simulink model "opv_receiver_HDL_coder_input_ISRO_Paper"  (R2023a)
settings: Solver=FixedStepDiscrete  StartTime=0.0  StopTime=0.01*(samples_per_frame/sample_rate)  RelTol=1e-3
values from neighbouring files (symbols this model uses):
  bit_rate = bits_per_symbol*symbol_rate    (= 54200)    [opv.m]
  bits_per_symbol = 2    [opv.m]
  carrier_frequency = carrier_frequency_multiple_ceil*(orthogonal_frequency)    [opv.m]
  device_clock = 245.76e6    (= 245760000)    [opv.m]
  orthogonal_frequency = 1/(4*bit_period)    (= 13550)    [opv.m]
  symbol_rate = 27100    [opv.m]
libraries: dspsrcs4 x4, simulink_extras x2, hdlsllib x1, commsrccod2 x1, dsphdlsigops2 x1, commrandsrc3 x1
settings Model: Creator=matt  LastModifiedBy=matt
settings OptimizationCC: BlockReduction=off  ConditionallyExecuteInputs=off  DefaultParameterBehavior=Inlined
settings DebuggingCC: AlgebraicLoopMsg=error
settings HardwareCC: ProdBitPerPointer=32  ProdBitPerSizeT=32  ProdBitPerPtrDiffT=32  ProdLargestAtomicFloat=None  ProdIntDivRoundTo=Undefined  ProdEndianess=Unspecified  ProdWordSize=32  ProdHWDeviceType=ASIC/FPGA->ASIC/FPGA  TargetBitPerLong=64  TargetBitPerPointer=64  TargetBitPerSizeT=64  TargetBitPerPtrDiffT=64  TargetLongLongMode=on  TargetIntDivRoundTo=Zero  TargetEndianess=LittleEndian  TargetWordSize=64  TargetHWDeviceType=Custom Processor->MATLAB Host Computer  ProdEqTarget=off

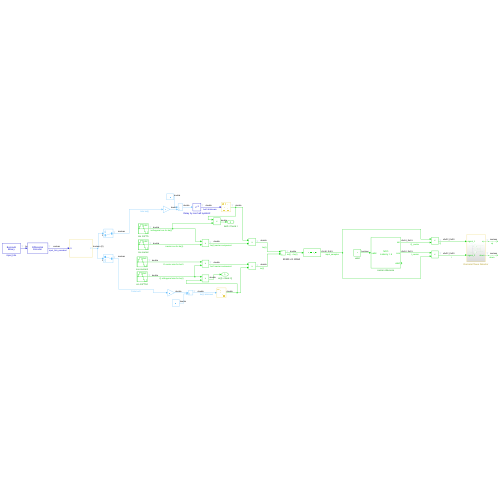
[thumbnail: Simulink's stored preview of the top-level diagram]
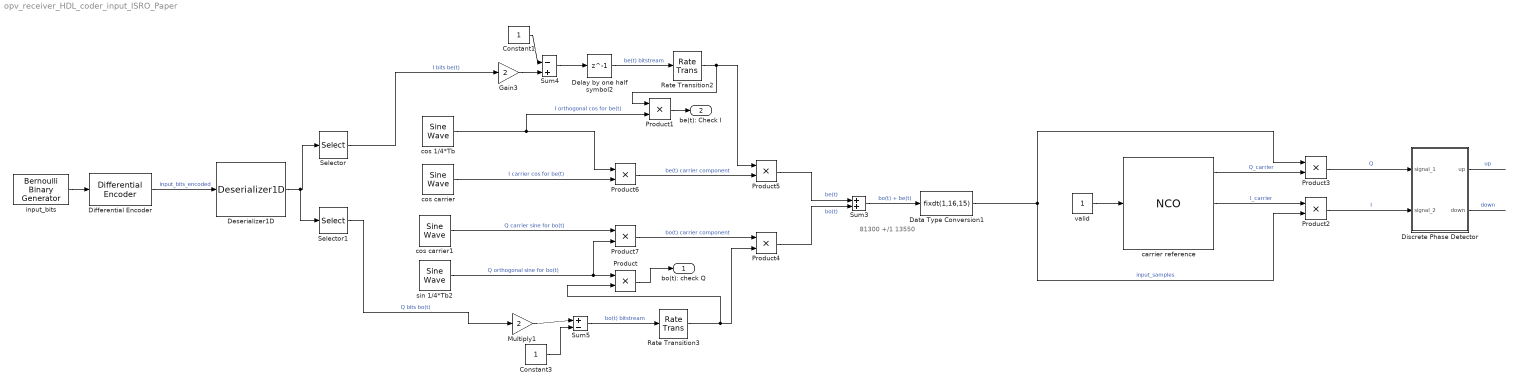
== system opv_receiver_HDL_coder_input_ISRO_Paper ==
  note: 81300 +/1 13550
  Constant1 : Constant  OutDataTypeStr=double  SampleTime=1/symbol_rate
  Constant3 : Constant  OutDataTypeStr=double  SampleTime=1/symbol_rate
  Data Type Conversion1 : DataTypeConversion  OutDataTypeStr=fixdt(1,16,15)  SaturateOnIntegerOverflow=off  RndMeth=Floor
  Delay by one half symbol2 : Delay  DelayLength=1  SampleTime=1/(bits_per_symbol*symbol_rate)
  Deserializer1D : hdlsllib/HDL Operations/Deserializer1D  Ratio=2  IdleCycles=0  InitialCondition=0  startIn=off  validIn=off  validOut=off  inputDataDimensions=-1  inputSampleTime=-1  inputSignalType=auto
  Differential Encoder : commsrccod2/Differential Encoder  InitCond=0
  Discrete Phase Detector : Subsystem
  Gain3 : Gain  Gain=2  OutDataTypeStr=double
  Multiply1 : Gain  Gain=2  OutDataTypeStr=double
  Product{,1..5} (6 alike) : Product
  Product6 : Product  OutDataTypeStr=double
  Product7 : Product  OutDataTypeStr=double
  Rate Transition2 : RateTransition  Deterministic=off  OutPortSampleTimeMultiple=device_clock/symbol_rate  OutPortSampleTime=1/device_clock
  Rate Transition3 : RateTransition  Deterministic=off  OutPortSampleTimeMultiple=device_clock/symbol_rate  OutPortSampleTime=1/device_clock
  Selector : Selector  InputPortWidth=2  IndexOptions=Index vector (dialog)  Indices=[2:2]  OutputSizes=1
  Selector1 : Selector  InputPortWidth=2  IndexOptions=Index vector (dialog)  Indices=[1:1]  OutputSizes=1
  Sum3 : Sum  AccumDataTypeStr=double
  Sum4 : Sum  Inputs=|-+  AccumDataTypeStr=double
  Sum5 : Sum  Inputs=|+-  AccumDataTypeStr=double
  carrier reference : dsphdlsigops2/NCO  PhaseIncrementSource=Property  PhaseIncrement=phase_increment_carrier  PhaseOffsetSource=Property  PhaseOffset=0  DitherSource=None  NumDitherBits=16  SamplesPerFrame=1  LUTCompress=on  ResetAction=off  Waveform=Sine and cosine  PhasePort=off  SimulateUsing=Code generation  AccumulatorWL=32  PhaseQuantization=on  NumQuantizerAccumulatorBits=19  OutputDataType=Binary point scaling  OutputWL=16  OutputFL=15
      settings: LibrarySourceBlock=dsphdlsrcs2/NCO
  cos 1/4*Tb : dspsrcs4/Sine Wave  Amplitude=1  Frequency=orthogonal_frequency  Phase=pi/2  SampleMode=Discrete  OutComplex=Real  CompMethod=Trigonometric fcn  TableSize=Speed  SampleTime=1/device_clock  SamplesPerFrame=1  ResetState=Restart at time zero  OutputFrames=off  dataType=double  wordLen=16  udDataType=sfix(16)  fracBitsMode=User-defined  numFracBits=0  OutDataTypeStr=double  LastOutDataTypeStr=double
  cos carrier : dspsrcs4/Sine Wave  Amplitude=1  Frequency=carrier_frequency  Phase=pi/2  SampleMode=Discrete  OutComplex=Real  CompMethod=Trigonometric fcn  TableSize=Speed  SampleTime=1/device_clock  SamplesPerFrame=1  ResetState=Restart at time zero  OutputFrames=off  dataType=double  wordLen=16  udDataType=sfix(16)  fracBitsMode=User-defined  numFracBits=0  OutDataTypeStr=double  LastOutDataTypeStr=double
  cos carrier1 : dspsrcs4/Sine Wave  Amplitude=1  Frequency=carrier_frequency  Phase=0  SampleMode=Discrete  OutComplex=Real  CompMethod=Trigonometric fcn  TableSize=Speed  SampleTime=1/device_clock  SamplesPerFrame=1  ResetState=Restart at time zero  OutputFrames=off  dataType=double  wordLen=16  udDataType=sfix(16)  fracBitsMode=User-defined  numFracBits=0  OutDataTypeStr=double  LastOutDataTypeStr=double
  input_bits : commrandsrc3/Bernoulli Binary Generator  ProbabilityOfZero=0.5  SeedSource=Auto  Seed=0  SampleTime=1/(bit_rate)  SamplesPerFrame=1  OutputDataType=boolean  SimulateUsing=Interpreted execution
  sin 1/4*Tb2 : dspsrcs4/Sine Wave  Amplitude=1  Frequency=orthogonal_frequency  Phase=0  SampleMode=Discrete  OutComplex=Real  CompMethod=Trigonometric fcn  TableSize=Speed  SampleTime=1/device_clock  SamplesPerFrame=1  ResetState=Restart at time zero  OutputFrames=off  dataType=double  wordLen=16  udDataType=sfix(16)  fracBitsMode=User-defined  numFracBits=0  OutDataTypeStr=double  LastOutDataTypeStr=double
  valid : Constant  OutDataTypeStr=boolean  SampleTime=1/device_clock
  bo(t): check Q : Outport
  be(t): Check I : Outport  Port=2
  wires:
  sin 1/4*Tb2/1 -> Product7/2, Product/1  "Q orthogonal sine for bo(t)"
  cos carrier1/1 -> Product7/1  "Q carrier sine for bo(t)"
  Sum3/1 -> Data Type Conversion1/1  "bo(t) + be(t)"
  Product6/1 -> Product5/2  "be(t) carrier component"
  Product7/1 -> Product4/1  "bo(t) carrier component"
  cos 1/4*Tb/1 -> Product6/1, Product1/2  "I orthogonal cos for be(t)"
  cos carrier/1 -> Product6/2  "I carrier cos for be(t)"
  Data Type Conversion1/1 -> Product3/1, Product2/2  "input_samples"
  Multiply1/1 -> Sum5/1
  Constant3/1 -> Sum5/2
  Product4/1 -> Sum3/2  "bo(t)"
  Product5/1 -> Sum3/1  "be(t)"
  Sum4/1 -> Delay by one half symbol2/1
  Rate Transition2/1 -> Product5/1, Product1/1
  Rate Transition3/1 -> Product/2, Product4/2
  Sum5/1 -> Rate Transition3/1  "bo(t) bitstream"
  Gain3/1 -> Sum4/2
  Constant1/1 -> Sum4/1
  Product/1 -> bo(t): check Q/1
  Product1/1 -> be(t): Check I/1
  Delay by one half symbol2/1 -> Rate Transition2/1  "be(t) bitstream"
  input_bits/1 -> Differential Encoder/1
  Differential Encoder/1 -> Deserializer1D/1  "input_bits_encoded"
  Selector/1 -> Gain3/1  "I bits be(t)"
  Selector1/1 -> Multiply1/1  "Q bits bo(t)"
  Deserializer1D/1 -> Selector1/1, Selector/1
  valid/1 -> carrier reference/1
  carrier reference/2 -> Product2/1  "I_carrier"
  carrier reference/1 -> Product3/2  "Q_carrier"
  Product3/1 -> Discrete Phase Detector/1(signal_1)  "Q"
  Product2/1 -> Discrete Phase Detector/2(signal_2)  "I"
  Discrete Phase Detector/1(up) -> ?  "up"
  Discrete Phase Detector/2(down) -> ?  "down"

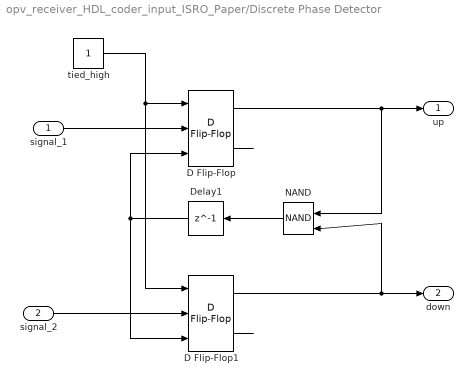
== system opv_receiver_HDL_coder_input_ISRO_Paper/Discrete Phase Detector ==
  signal_1 : Inport
  signal_2 : Inport  Port=2
  D Flip-Flop : simulink_extras/Flip Flops/D Flip-Flop
  D Flip-Flop1 : simulink_extras/Flip Flops/D Flip-Flop
  Delay1 : Delay  DelayLength=1
  NAND : Logic  Operator=NAND  IconShape=distinctive  AllPortsSameDT=off  OutDataTypeStr=boolean
  tied_high : Constant  OutDataTypeStr=boolean  SampleTime=1/symbol_rate
  up : Outport
  down : Outport  Port=2
  wires:
  signal_1/1 -> D Flip-Flop/2
  signal_2/1 -> D Flip-Flop1/2
  NAND/1 -> Delay1/1
  tied_high/1 -> D Flip-Flop1/1, D Flip-Flop/1
  D Flip-Flop/2 -> ?
  D Flip-Flop1/2 -> ?
  D Flip-Flop/1 -> up/1, NAND/1
  D Flip-Flop1/1 -> down/1, NAND/2
  Delay1/1 -> D Flip-Flop1/3, D Flip-Flop/3
